simulink model "LandingGear"  (R2018b)
settings: Solver=FixedStepAuto  StartTime=0.0  StopTime=inf  RelTol=1e-3
libraries: sldrtlib x1
settings Model: Creator=Khrisna Adi Kamarga  LastModifiedBy=Khrisna Adi Kamarga

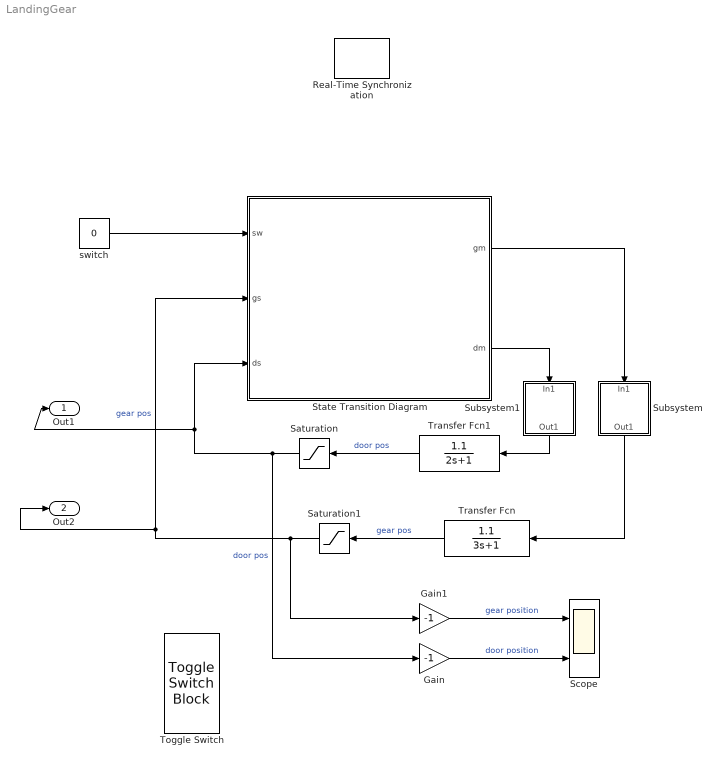
== system LandingGear ==
  Gain : Gain  Gain=-1
  Gain1 : Gain  Gain=-1
  Real-Time Synchronization : sldrtlib/Real-Time Synchronization  SampleTime=0.1  MaxMissedTicks=10  ShowMissedTicks=off  YieldWhenWaiting=off
  Saturation : Saturate  UpperLimit=1  LowerLimit=-1
  Saturation1 : Saturate  UpperLimit=1  LowerLimit=-1
  Scope : Scope  NumInputPorts=2
  State Transition Diagram : Stateflow chart  TreatAsAtomicUnit=on
  Subsystem : Subsystem
  Subsystem1 : Subsystem
  Toggle Switch : ToggleSwitchBlock  WebBlockId=3
      settings: Values={{'raise', 'lower'}, [0 1]}
  Transfer Fcn : TransferFcn  Numerator=[1.1]  Denominator=[3 1]
  Transfer Fcn1 : TransferFcn  Numerator=[1.1]  Denominator=[2 1]
  switch : Constant  Value=0
  Out1 : Outport  SignalName=door pos
  Out2 : Outport  Port=2  SignalName=gear pos
  wires:
  switch/1 -> State Transition Diagram/1(sw)
  Transfer Fcn/1 -> Saturation1/1  "gear pos"
  Transfer Fcn1/1 -> Saturation/1  "door pos"
  Saturation/1 -> Gain/1, State Transition Diagram/3(ds), Out1/1  "door pos"
  Saturation1/1 -> Gain1/1, State Transition Diagram/2(gs), Out2/1  "gear pos"
  Subsystem/1(Out1) -> Transfer Fcn/1
  State Transition Diagram/1(gm) -> Subsystem/1(In1)
  State Transition Diagram/2(dm) -> Subsystem1/1(In1)
  Subsystem1/1(Out1) -> Transfer Fcn1/1
  Gain/1 -> Scope/2  "door position"
  Gain1/1 -> Scope/1  "gear position"

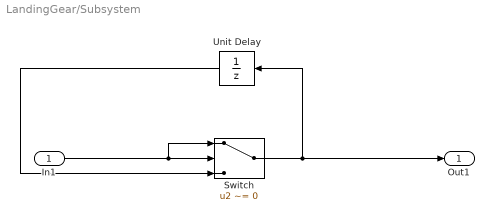
== system LandingGear/Subsystem ==
  In1 : Inport
  Switch : Switch  Criteria=u2 ~= 0
  Unit Delay : UnitDelay  SampleTime=-1
  Out1 : Outport
  wires:
  In1/1 -> Switch/1, Switch/2
  Switch/1 -> Unit Delay/1, Out1/1
  Unit Delay/1 -> Switch/3

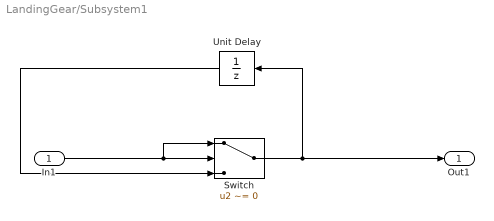
== system LandingGear/Subsystem1 ==
  In1 : Inport
  Switch : Switch  Criteria=u2 ~= 0
  Unit Delay : UnitDelay  SampleTime=-1
  Out1 : Outport
  wires:
  In1/1 -> Switch/1, Switch/2
  Switch/1 -> Unit Delay/1, Out1/1
  Unit Delay/1 -> Switch/3

== stateflow chart LandingGear/State Transition Diagram ==
  note: sw:
      | 	raise = 0
      | 	lower = 1
      | gs:
      | 	bottom = 1
      | 	top = -1
      | 	other = between
      | ds:
      | 	opened = 1
      | 	closed = -1
      | gm:
      | 	raising = -1
      | 	lowering = 1
      | 	off = 0
      | dm:
      | 	opening = 1
      | 	closing = -1
      | 	off = 0
  state GS
  state DMC
  state DMO
  state GMU
  state GMD
  state GL
  (default) -> GS
  DMC -> GS [order 1] : [ds == -1]{dm = 0}
  GS -> DMO : [sw == 1]{dm = 1}
  DMC -> DMO [order 2] : [sw  == 1]{dm = 1}
  DMO -> DMC [order 2] : [sw == 0]{dm = -1}
  GMU -> DMC [order 1] : [gs == -1]{gm = 0; dm = -1}
  DMO -> GMD [order 1] : [ds == 1]{gm = 1; dm = 0}
  GMU -> GMD [order 2] : [sw == 1]{gm = 1}
  GMD -> GMU [order 2] : [sw == 0]{gm = -1}
  GL -> GMU : [sw == 0]{gm = -1}
  GMD -> GL [order 1] : [gs == 1]{gm = 0}
  data: sw input; gs input; ds input; gm output =0; dm output =0
